simulink model "Control_v6_LQR_2020b"  (R2020b)
settings: Solver=FixedStepAuto  StartTime=0.0  StopTime=t_sim  FixedStep=TimeStep  RelTol=1e-3
values from neighbouring files (symbols this model uses):
  R = [ 1    0            0;         0    cos(alpha)  -sin(alpha);         0    sin(alpha)   cos(alpha)]    [main_SCA_v3.m]    (also in main_SCA_v3_alt.m; main_SCA_v4_LQR.m; main_SCA_v5.m)
  Use_IGRF = 0    [main_SCA.m]    (also in main_SCA_v3.m; main_SCA_v3_alt.m; main_SCA_v4_LQR.m; main_SCA_v5.m = 1)
undefined symbols (not defined in the file or in its folder): att, C, date, deg, DiscIntNeverNeededParam, IonSataero, Isat_inverse, km, orbit, Q, rad, s, sat
libraries: vrlib x23, aerolibutil x16, dspmathops x15, aerolibconvert2 x14, sharedtransform x13, simulink x4, simulink_extras x2, aerolibatmos2 x1, DipoleModel x1, aerolibobsolete x1, sharedutil x1, aerolibcelestial x1
(part 4 of 4)

== matlab function Control_v6_LQR_2020b/Attitude Controller/LQR (nominal command)/Inverse nxn matrix1 ==
  data: u input; y output
function y = fcn(u)

y = inv(u);

== matlab function Control_v6_LQR_2020b/Time propagator/MATLAB Function ==
  data: t input; Y output; DOY output; S output
function [Y, DOY, S] = DOY(t)
Y = 2022 + fix(t/31557600);
DOY = 1+fix((t-floor(t/31557600)*31557600)/86400);
S = t - fix(t/31557600)*31557600 - (DOY-1)*86400;

== matlab function Control_v6_LQR_2020b/Attitude Controller/LQR (nominal command)/Inverse nxn matrix2 ==
  data: u input; y output
function y = fcn(u)

y = inv(u);

== matlab function Control_v6_LQR_2020b/Attitude Controller/LQR (nominal command)/Is the system observable? ==
  data: Gv input; y output
function y = fcn(Gv)

Gv_rank = rank(Gv);

if Gv_rank == 6
    y = "the system is observable";
else
    y = "the system isn't observable";
end

== matlab function Control_v6_LQR_2020b/Reference/q_drag/"Avoids" sign change should be improved/MATLAB Function ==
  data: u1 input; y output; u2 input
function y  = fcn(u1, u2)
s=dot(sign(u1),sign(u2));
if sign(s)<0
    y=1;
else
    y=0;
end
end

== matlab function Control_v6_LQR_2020b/Attitude Controller/LQR (nominal command)/returns the feedback gain that are used ==
  data: K input; k_qe1 output; k_qe2 output; k_qe3 output; k_w1 output; k_w2 output; k_w3 output
function [k_qe1,k_qe2,k_qe3,k_w1,k_w2,k_w3] = fcn(K)

k_qe1 = K(1);
k_qe2 = K(5);
k_qe3 = K(9);
k_w1 = K(10);
k_w2 = K(14);
k_w3 = K(18);

== matlab function Control_v6_LQR_2020b/Reference/q_drag/"Avoids" sign change should be improved/MATLAB Function1 ==
  data: u input; y output
function y = fcn(u)

y = mod(u,2);

== matlab function Control_v6_LQR_2020b/Disturbance Torques/Aerodynamic Model/Get Density/ECI To LLA ==
  data: X_ECEF input; h output; lat output; long output
function [h, lat, long] = fcn(X_ECEF)
    h = 0;
    lat = 0;
    long = 0;
[lat, long, h] = ecef2geod(X_ECEF(1),X_ECEF(2),X_ECEF(3));

== matlab function Control_v6_LQR_2020b/Reference/q_orbital/"Avoids" sign change should be improved/MATLAB Function ==
  data: u1 input; y output; u2 input
function y  = fcn(u1, u2)
s=dot(sign(u1),sign(u2));
if sign(s)<0
    y=1;
else
    y=0;
end
end

== matlab function Control_v6_LQR_2020b/Reference/q_orbital/"Avoids" sign change should be improved/MATLAB Function1 ==
  data: u input; y output
function y = fcn(u)

y = mod(u,2);

== matlab function Control_v6_LQR_2020b/Reference/q_retrograde/"Avoids" sign change should be improved/MATLAB Function ==
  data: u1 input; y output; u2 input
function y  = fcn(u1, u2)
s=dot(sign(u1),sign(u2));
if sign(s)<0
    y=1;
else
    y=0;
end
end

== matlab function Control_v6_LQR_2020b/Reference/q_retrograde/"Avoids" sign change should be improved/MATLAB Function1 ==
  data: u input; y output
function y = fcn(u)

y = mod(u,2);

== matlab function Control_v6_LQR_2020b/Reference/q_sun_sun/"Avoids" sign change should be improved/MATLAB Function ==
  data: u1 input; y output; u2 input
function y  = fcn(u1, u2)
s=dot(sign(u1),sign(u2));
if sign(s)<0
    y=1;
else
    y=0;
end
end

== matlab function Control_v6_LQR_2020b/Reference/q_sun_sun/"Avoids" sign change should be improved/MATLAB Function1 ==
  data: u input; y output
function y = fcn(u)

y = mod(u,2);

== matlab function Control_v6_LQR_2020b/Reference/q_sun_aero/"Avoids" sign change should be improved/MATLAB Function ==
  data: u1 input; y output; u2 input
function y  = fcn(u1, u2)
s=dot(sign(u1),sign(u2));
if sign(s)<0
    y=1;
else
    y=0;
end
end

== matlab function Control_v6_LQR_2020b/Reference/q_sun_aero/"Avoids" sign change should be improved/MATLAB Function1 ==
  data: u input; y output
function y = fcn(u)

y = mod(u,2);

== matlab function Control_v6_LQR_2020b/Reference/q_sun_drag/"Avoids" sign change should be improved/MATLAB Function ==
  data: u1 input; y output; u2 input
function y  = fcn(u1, u2)
s=dot(sign(u1),sign(u2));
if sign(s)<0
    y=1;
else
    y=0;
end
end

== matlab function Control_v6_LQR_2020b/Reference/q_sun_drag/"Avoids" sign change should be improved/MATLAB Function1 ==
  data: u input; y output
function y = fcn(u)

y = mod(u,2);

== matlab function Control_v6_LQR_2020b/Initialize Function/orb2rv ==
  data: a input; r output; e input; i input; O input; o input; nu input; v output; truLon input; argLat input; lonPer input
%----------------------- Begin Code Sequence -----------------------------%
% Purpose:                                                                %
% Convert a given set of Keplerian Orbital Elements to state vectors in   %
% in the ECI frame of reference                                           %
%                                                                         %
%-------------------------------------------------------------------------%
%                                                                         %
% Inputs:                                                                 %
%-------- 
%a                      [1 x N]                         Semimajor axis
%                                                       (km)
%
%e                      [1 x N]                         Eccentricity Magnitude
%                                                       (unitless)
%
%i                      [1 x N]                         inclination
%                                                       (radians)
%
%O                      [1 x N]                         Right Ascention of
%                                                       the ascending node
%                                                       (radians)
%
%o                      [1 x N]                         Argument of perigee
%                                                       (radians)
%
%nu                     [1 x N]                         True Anomaly
%                                                       (radians)
%
%truLon                 [1 x N]                         True Longitude
%                                                       (radians)
%
%argLat                 [1 x N]                         Argument of Latitude
%                                                       (radians)
%
%lonPer                 [1 x N]                         Longitude of Periapse
%                                                       (radians)
%
%mu                     double                          Gravitational Constant
%                                                       Defaults to Earth if
%                                                       not specified
%
% Outputs:
%---------                                                                %
%r_ECI                  [3 x N]                         Position Vector in
%                                                       ECI coordinate
%                                                       frame of reference
%
%v_ECI                  [3 x N]                         Velocity vector in
%                                                       ECI coordinate
%                                                       frame of reference
%
% References:
%-------------
%Vallado,D. Fundamentals of Astrodynamics and Applications. 2007.
%
% Function Dependencies:
%------------------
%None
%------------------------------------------------------------------       %
% Programed by Darin Koblick  03-04-2012                                  %
%------------------------------------------------------------------       %
function [r,v] = orb2rv(a,e,i,O,o,nu,truLon,argLat,lonPer)
mu = 398600.4418;
%Make all inputs consistent w/ dimensions
a = a(:); e = e(:); i = i(:); O = O(:); o = o(:); nu = nu(:);
if e<1
    p=a*(1-e*e);
else
    p=2*a;
end
ietol = 1e-8;
idx = e < ietol & mod(i,pi) < ietol;
if any(idx); o(idx) = 0; O(idx) = 0; nu(idx) = truLon(idx); end
idx = e < ietol & mod(i,pi) > ietol;
if any(idx); o(idx) = 0; nu(idx) = argLat(idx); end
idx = e > ietol & mod(i,pi) < ietol;
if any(idx); O(idx) = 0; o(idx) = lonPer(idx); end
%Find rPQW and vPQW
rPQW = cat(2,p.*cos(nu)./(1 +e.*cos(nu)),p.*sin(nu)./(1+e.*cos(nu)),zeros(size(nu)));
vPQW = cat(2,-sqrt(mu./p).*sin(nu),sqrt(mu./p).*(e+cos(nu)),zeros(size(nu)));
%Create Transformation Matrix
PQW2IJK = NaN(3,3,size(p,1));
cO = cos(O); sO = sin(O); co = cos(o); so = sin(o); ci = cos(i); si = sin(i);
PQW2IJK(1,1,:) = cO.*co-sO.*so.*ci; PQW2IJK(1,2,:) = -cO.*so-sO.*co.*ci; PQW2IJK(1,3,:) = sO.*si;
PQW2IJK(2,1,:) = sO.*co+cO.*so.*ci; PQW2IJK(2,2,:) = -sO.*so+cO.*co.*ci; PQW2IJK(2,3,:) = -cO.*si;
PQW2IJK(3,1,:) = so.*si;            PQW2IJK(3,2,:) = co.*si;             PQW2IJK(3,3,:) = ci;
%Transform rPQW and vPQW to rECI and vECI
r = multiDimMatrixMultiply(PQW2IJK,rPQW)';  
v = multiDimMatrixMultiply(PQW2IJK,vPQW)';
end
function c = multiDimMatrixMultiply(a,b)
c = NaN(size(b));
c(:,1) = sum(bsxfun(@times,a(1,:,:),permute(b,[3 2 1])),2);
c(:,2) = sum(bsxfun(@times,a(2,:,:),permute(b,[3 2 1])),2);
c(:,3) = sum(bsxfun(@times,a(3,:,:),permute(b,[3 2 1])),2);
end

== matlab function Control_v6_LQR_2020b/Disturbance Torques/Aerodynamic Model/Get Density/MATLAB Function2 ==
  data: u input; y output
function y = fcn(u)
y = u(6);

== matlab function Control_v6_LQR_2020b/IGRF Computation block/MATLAB Function ==
  data: u input; y output
function y = fcn(u)
%#codegen

y = norm(u);

== matlab function Control_v6_LQR_2020b/IGRF Computation block/ECI To LLA ==
  data: X_ECEF input; h output; lat output; long output
function [h, lat, long] = fcn(X_ECEF)
    h = 0;
    lat = 0;
    long = 0;
[lat, long, h] = ecef2geod(X_ECEF(1),X_ECEF(2),X_ECEF(3));

== matlab function Control_v6_LQR_2020b/Disturbance Torques/Aerodynamic Model/Calculate - Az & El Angle/MATLAB Function ==
  data: x input; elevation output; y input; z input
function elevation = fcn(x,y,z)

elevation = z/sqrt(x^2 + y^2 + z^2);

== matlab function Control_v6_LQR_2020b/Time propagator/UTC to JD ==
  data: Time_UTC input; JD output
function JD = fcn(Time_UTC)

% JD = juliandate(Time_UTC);
JD = Dt2jD(Time_UTC);

== matlab function Control_v6_LQR_2020b/Time propagator/JD to UTC ==
  data: JD input; Time_UTC output
function Time_UTC = fcn(JD)
    coder.extrinsic('datetime','datevec');
    Time_UTC = [0,0,0,0,0,0];
Time_UTC =  datevec(datetime(JD,'convertfrom','juliandate'));

== matlab function Control_v6_LQR_2020b/Thruster activation/MATLAB Function ==
  data: u input; y output
function y = fcn(u)
% t0 less or equal than waiting time between 2 thrusts
% or 
% sat.thruster.firstimpulse <= sat.thruster.wait

time=u(1);
duration=u(2);
t0=u(3);
wait=u(4);
N=u(5)-1;
boolean=0;
booleant=0;

if (time<t0)
    boolean=0;
end

if (time>=t0)
        m=fix(time/(duration+wait));
        if (m<=N)&&((t0+m*(duration+wait)<time)&&(time<(t0+m*(duration+wait)+duration)))
            boolean=1;
        end
        
end

y = booleant~=boolean;

== matlab function Control_v6_LQR_2020b/Attitude Controller/RW power // saturation/Steady state Power consumption ==
  data: RW1 input; WP1 output; RW2 input; RW3 input; RW4 input; WP2 output; WP3 output; WP4 output
function [WP1,WP2,WP3,WP4] = fcn(RW1,RW2,RW3,RW4)

WP1 = 0.1414*RW1 - 68.988;
WP2 = 0.1414*RW2 - 68.988;
WP3 = 0.1414*RW3 - 68.988;
WP4 = 0.1414*RW4 - 68.988;
